simulink model "hw2_SISO_2_3_chann_final"  (R2023b)
settings: Solver=ode15s  StartTime=0.0  StopTime=4  FixedStep=0.001  RelTol=1e-3
values from neighbouring files (symbols this model uses):
  A = 1    [hw1_four_channel_bilateral_teleoperation_params.m]    (also in hw2_2_3_channel_bilateral_teleoperation_params.m; hw3_scattering_teleop_FP_params.m = 1.5; hw3_scattering_teleop_PP_params.m; hw4_tank_FP_params.m)
  Be = 100    [hw1_four_channel_bilateral_teleoperation_params.m]    (also in hw2_2_3_channel_bilateral_teleoperation_params.m; hw3_scattering_teleop_FP_params.m; hw3_scattering_teleop_PP_params.m; hw4_tank_FP_params.m)
  Bh = 1    [hw1_four_channel_bilateral_teleoperation_params.m]    (also in hw2_2_3_channel_bilateral_teleoperation_params.m; hw3_scattering_teleop_FP_params.m; hw3_scattering_teleop_PP_params.m; hw4_tank_FP_params.m)
  Bm = 20*0.8    (= 16)    [hw1_four_channel_bilateral_teleoperation_params.m]    (also in hw2_2_3_channel_bilateral_teleoperation_params.m; hw3_scattering_teleop_FP_params.m; hw3_scattering_teleop_PP_params.m; hw4_tank_FP_params.m = 32)
  Bs = 4*Bm    (= 64)    [hw1_four_channel_bilateral_teleoperation_params.m]    (also in hw2_2_3_channel_bilateral_teleoperation_params.m; hw3_scattering_teleop_FP_params.m; hw3_scattering_teleop_PP_params.m; hw4_tank_FP_params.m = 128)
  d = 0.02    [hw2_2_3_channel_bilateral_teleoperation_params.m]    (also in hw3_scattering_teleop_FP_params.m = 10; hw3_scattering_teleop_PP_params.m = 10; hw4_tank_FP_params.m = 10; hw4_tank_PP_params.m = 10)
  Dh = 20*0.8    (= 16)    [hw1_four_channel_bilateral_teleoperation_params.m]    (also in hw2_2_3_channel_bilateral_teleoperation_params.m; hw3_scattering_teleop_FP_params.m; hw3_scattering_teleop_PP_params.m; hw4_tank_FP_params.m)
  Dm = 0    [hw1_four_channel_bilateral_teleoperation_params.m]    (also in hw2_2_3_channel_bilateral_teleoperation_params.m; hw3_scattering_teleop_FP_params.m = 5; hw3_scattering_teleop_PP_params.m; hw4_tank_FP_params.m)
  Ds = 0    [hw1_four_channel_bilateral_teleoperation_params.m]    (also in hw2_2_3_channel_bilateral_teleoperation_params.m; hw3_scattering_teleop_FP_params.m; hw3_scattering_teleop_PP_params.m; hw4_tank_FP_params.m)
  Fc = 1    [hw1_four_channel_bilateral_teleoperation_params.m]    (also in hw2_2_3_channel_bilateral_teleoperation_params.m; hw3_scattering_teleop_FP_params.m; hw3_scattering_teleop_PP_params.m; hw4_tank_FP_params.m)
  Flp = 0.5    [hw1_four_channel_bilateral_teleoperation_params.m]    (also in hw2_2_3_channel_bilateral_teleoperation_params.m; hw3_scattering_teleop_FP_params.m = 0.01; hw3_scattering_teleop_PP_params.m = 0.01; hw4_tank_FP_params.m = 1)
  Jh = 1    [hw1_four_channel_bilateral_teleoperation_params.m]    (also in hw2_2_3_channel_bilateral_teleoperation_params.m; hw3_scattering_teleop_FP_params.m; hw3_scattering_teleop_PP_params.m; hw4_tank_FP_params.m)
  Ke = 200    [hw1_four_channel_bilateral_teleoperation_params.m]    (also in hw2_2_3_channel_bilateral_teleoperation_params.m; hw3_scattering_teleop_FP_params.m; hw3_scattering_teleop_PP_params.m; hw4_tank_FP_params.m)
  Km = 10*1    (= 10)    [hw1_four_channel_bilateral_teleoperation_params.m]    (also in hw2_2_3_channel_bilateral_teleoperation_params.m; hw3_scattering_teleop_FP_params.m; hw3_scattering_teleop_PP_params.m; hw4_tank_FP_params.m)
  Ks = 4*Km    (= 40)    [hw1_four_channel_bilateral_teleoperation_params.m]    (also in hw2_2_3_channel_bilateral_teleoperation_params.m; hw3_scattering_teleop_FP_params.m; hw3_scattering_teleop_PP_params.m; hw4_tank_FP_params.m)
  Mm = 0.5    [hw1_four_channel_bilateral_teleoperation_params.m]    (also in hw2_2_3_channel_bilateral_teleoperation_params.m; hw3_scattering_teleop_FP_params.m; hw3_scattering_teleop_PP_params.m; hw4_tank_FP_params.m)
  Ms = 2    [hw1_four_channel_bilateral_teleoperation_params.m]    (also in hw2_2_3_channel_bilateral_teleoperation_params.m; hw3_scattering_teleop_FP_params.m; hw3_scattering_teleop_PP_params.m; hw4_tank_FP_params.m)
  Ph = 10*1    (= 10)    [hw1_four_channel_bilateral_teleoperation_params.m]    (also in hw2_2_3_channel_bilateral_teleoperation_params.m; hw3_scattering_teleop_FP_params.m; hw3_scattering_teleop_PP_params.m; hw4_tank_FP_params.m)
  xe = 0.7    [hw1_four_channel_bilateral_teleoperation_params.m]    (also in hw2_2_3_channel_bilateral_teleoperation_params.m = 1.5; hw3_scattering_teleop_FP_params.m = 1.5; hw3_scattering_teleop_PP_params.m = 1.5; hw4_tank_FP_params.m = 1.5)
settings Model: Creator=86180  LastModifiedBy=86180

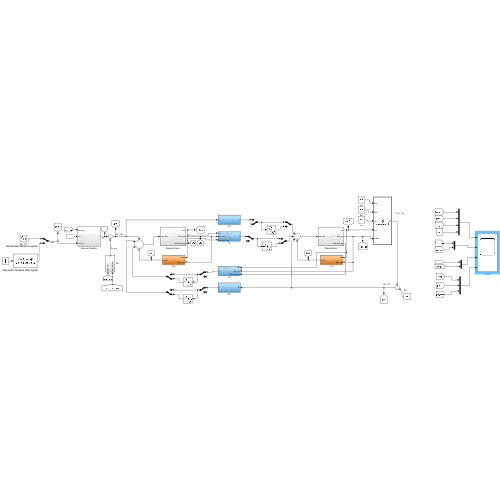
[thumbnail: Simulink's stored preview of the top-level diagram]
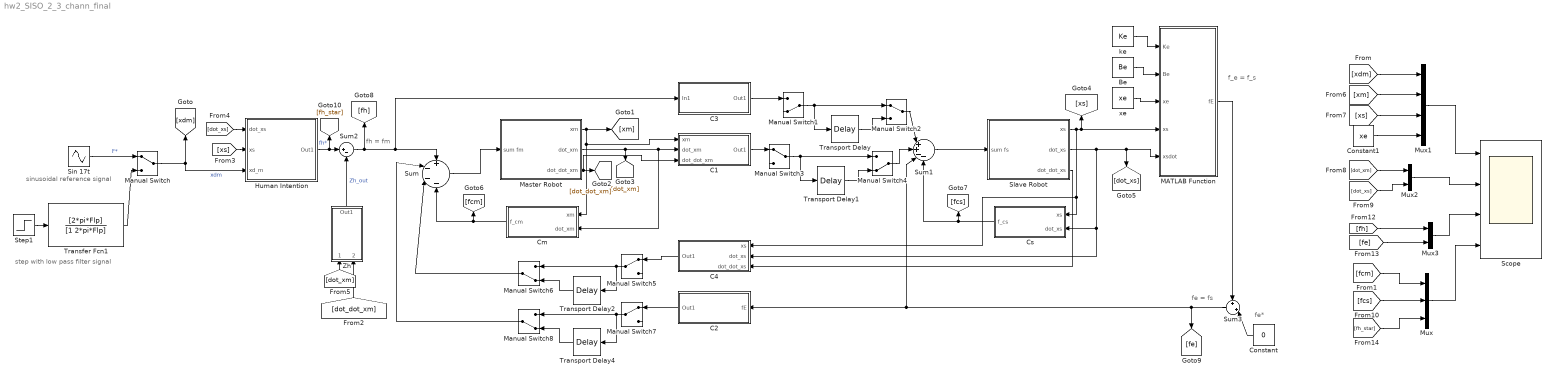
== system hw2_SISO_2_3_chann_final ==
  note: f_e = f_s
  note: fe*
  note: fe = fs
  note: fh = fm
  note: sinusoidal reference signal
  note: step with low pass filter signal
  Be : Constant  Value=Be
  C1 : Subsystem
  C2 : Subsystem
  C3 : Subsystem
  C4 : Subsystem
  Cm : Subsystem
  Constant : Constant  Value=0
  Constant1 : Constant  Value=xe
  Cs : Subsystem
  Human Intention : Subsystem
  MATLAB Function : MATLAB Function  TreatAsAtomicUnit=on
  Manual Switch{,2..3,5,7} (5 alike) : ManualSwitch
  Manual Switch{1,4,6,8} (4 alike) : ManualSwitch  CurrentSetting=0
  Master Robot : Subsystem
  Mux : Mux  Inputs=3
  Mux1 : Mux
  Mux2 : Mux  Inputs=2
  Mux3 : Mux  Inputs=2
  Scope : Scope  NumInputPorts=4
  Sin 17t : Sin  Amplitude=A  Frequency=2*pi*Fc  SampleTime=0
  Slave Robot : Subsystem
  Step1 : Step  Time=0.5  After=A  SampleTime=0
  Sum : Sum  Inputs=+---
  Sum1 : Sum  Inputs=|++--
  Sum2 : Sum  Inputs=|+-
  Sum3 : Sum  Inputs=+|+|
  Transfer Fcn1 : TransferFcn  Numerator=[2*pi*Flp]  Denominator=[1 2*pi*Flp]
  Transport Delay{,1..2,4} (4 alike) : TransportDelay  DelayTime=d
  Zh : Subsystem
  ke : Constant  Value=Ke
  xe : Constant  Value=xe
  wires:
  Manual Switch/1 -> Human Intention/3(xd_m), [xdm]  "xdm"
  Zh/1(Out1) -> Sum2/2  "Zh_out"
  Transfer Fcn1/1 -> Manual Switch/2
  Human Intention/1(Out1) -> [fh_star], Sum2/1  "fh*"
  Sin 17t/1 -> Manual Switch/1  "F*"
  Step1/1 -> Transfer Fcn1/1
  ke/1 -> MATLAB Function/1(Ke)
  xe/1 -> MATLAB Function/3(xe)
  Slave Robot/1(xs) -> Cs/1(xs), C4/1(xs), MATLAB Function/4(xs), [xs]
  MATLAB Function/1(fE) -> Sum3/1
  Be/1 -> MATLAB Function/2(Be)
  Sum2/1 -> C3/1(In1), Sum/1, [fh]
  Master Robot/2(dot_xm) -> [dot_xm], C1/2(dot_xm), Cm/2(dot_xm)
  Cm/1(f_cm) -> [fcm], Sum/4
  Slave Robot/2(dot_xs) -> Cs/2(dot_xs), C4/2(dot_xs), [dot_xs], MATLAB Function/5(xsdot)
  Cs/1(f_cs) -> [fcs], Sum1/4
  Sum3/1 -> [fe], C2/1(fE), Sum1/3
  Constant/1 -> Sum3/2
  Master Robot/1(xm) -> C1/1(xm), Cm/1(xm), [xm]
  Master Robot/3(dot_dot_xm) -> C1/3(dot_dot_xm), [dot_dot_xm]
  [dot_dot_xm] -> Zh/2(dot_dot_xm)
  [xs] -> Human Intention/2(xs)
  [dot_xs] -> Human Intention/1(dot_xs)
  Sum/1 -> Master Robot/1(sum fm)
  [dot_xm] -> Zh/1(dot_xm)
  Sum1/1 -> Slave Robot/1(sum fs)
  Slave Robot/3(dot_dot_xs) -> C4/3(dot_dot_xs)
  Mux1/1 -> Scope/1
  Constant1/1 -> Mux1/4
  [fh] -> Mux3/1
  [dot_xs] -> Mux2/2
  Mux3/1 -> Scope/3
  [fe] -> Mux3/2
  [xm] -> Mux1/2
  [fcm] -> Mux/1
  [dot_xm] -> Mux2/1
  [fcs] -> Mux/2
  [xs] -> Mux1/3
  Mux2/1 -> Scope/2
  [xdm] -> Mux1/1
  Mux/1 -> Scope/4
  [fh_star] -> Mux/3
  Transport Delay/1 -> Manual Switch2/2
  C3/1(Out1) -> Manual Switch1/1
  Manual Switch1/1 -> Transport Delay/1, Manual Switch2/1
  Manual Switch2/1 -> Sum1/1
  Manual Switch3/1 -> Transport Delay1/1, Manual Switch4/1
  C1/1(Out1) -> Manual Switch3/1
  Transport Delay1/1 -> Manual Switch4/2
  Manual Switch4/1 -> Sum1/2
  Transport Delay2/1 -> Manual Switch6/2
  Manual Switch6/1 -> Sum/3
  Manual Switch5/1 -> Transport Delay2/1, Manual Switch6/1
  C4/1(Out1) -> Manual Switch5/1
  C2/1(Out1) -> Manual Switch7/1
  Manual Switch7/1 -> Transport Delay4/1, Manual Switch8/1
  Manual Switch8/1 -> Sum/2
  Transport Delay4/1 -> Manual Switch8/2

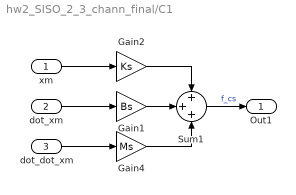
== system hw2_SISO_2_3_chann_final/C1 ==
  xm : Inport
  dot_xm : Inport  Port=2
  dot_dot_xm : Inport  Port=3
  Gain1 : Gain  Gain=Bs
  Gain2 : Gain  Gain=Ks
  Gain4 : Gain  Gain=Ms
  Sum1 : Sum  Inputs=+++
  Out1 : Outport
  wires:
  dot_xm/1 -> Gain1/1
  Gain1/1 -> Sum1/2
  dot_dot_xm/1 -> Gain4/1
  xm/1 -> Gain2/1
  Sum1/1 -> Out1/1  "f_cs"
  Gain2/1 -> Sum1/1
  Gain4/1 -> Sum1/3

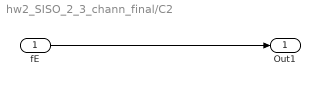
== system hw2_SISO_2_3_chann_final/C2 ==
  fE : Inport
  Out1 : Outport
  wires:
  fE/1 -> Out1/1

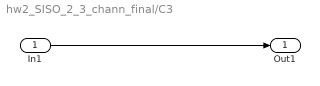
== system hw2_SISO_2_3_chann_final/C3 ==
  In1 : Inport
  Out1 : Outport
  wires:
  In1/1 -> Out1/1

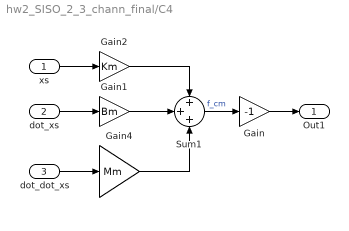
== system hw2_SISO_2_3_chann_final/C4 ==
  xs : Inport
  dot_xs : Inport  Port=2
  dot_dot_xs : Inport  Port=3
  Gain : Gain  Gain=-1
  Gain1 : Gain  Gain=Bm
  Gain2 : Gain  Gain=Km
  Gain4 : Gain  Gain=Mm
  Sum1 : Sum  Inputs=+++
  Out1 : Outport
  wires:
  Sum1/1 -> Gain/1  "f_cm"
  xs/1 -> Gain2/1
  dot_dot_xs/1 -> Gain4/1
  Gain1/1 -> Sum1/2
  Gain2/1 -> Sum1/1
  dot_xs/1 -> Gain1/1
  Gain4/1 -> Sum1/3
  Gain/1 -> Out1/1

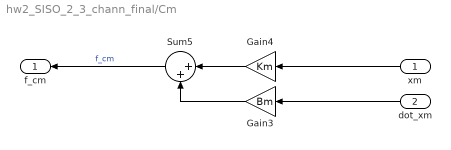
== system hw2_SISO_2_3_chann_final/Cm ==
  xm : Inport
  dot_xm : Inport  Port=2
  Gain3 : Gain  Gain=Bm
  Gain4 : Gain  Gain=Km
  Sum5 : Sum  Inputs=|++
  f_cm : Outport
  wires:
  Sum5/1 -> f_cm/1  "f_cm"
  Gain4/1 -> Sum5/1
  dot_xm/1 -> Gain3/1
  Gain3/1 -> Sum5/2
  xm/1 -> Gain4/1

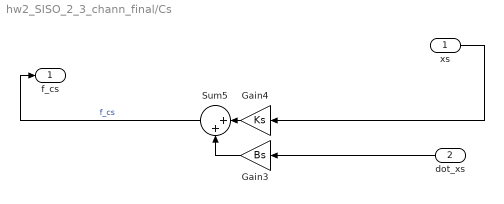
== system hw2_SISO_2_3_chann_final/Cs ==
  xs : Inport
  dot_xs : Inport  Port=2
  Gain3 : Gain  Gain=Bs
  Gain4 : Gain  Gain=Ks
  Sum5 : Sum  Inputs=|++
  f_cs : Outport
  wires:
  dot_xs/1 -> Gain3/1
  Sum5/1 -> f_cs/1  "f_cs"
  xs/1 -> Gain4/1
  Gain3/1 -> Sum5/2
  Gain4/1 -> Sum5/1

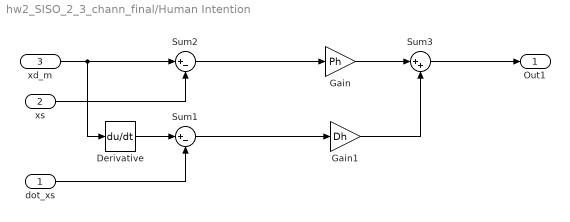
== system hw2_SISO_2_3_chann_final/Human Intention ==
  dot_xs : Inport
  xs : Inport  Port=2
  xd_m : Inport  Port=3
  Derivative : Derivative
  Gain : Gain  Gain=Ph
  Gain1 : Gain  Gain=Dh
  Sum1 : Sum  Inputs=|+-
  Sum2 : Sum  Inputs=|+-
  Sum3 : Sum  Inputs=|++
  Out1 : Outport
  wires:
  xs/1 -> Sum2/2
  dot_xs/1 -> Sum1/2
  Sum2/1 -> Gain/1
  Sum1/1 -> Gain1/1
  Gain1/1 -> Sum3/2
  Gain/1 -> Sum3/1
  Sum3/1 -> Out1/1
  xd_m/1 -> Derivative/1, Sum2/1
  Derivative/1 -> Sum1/1

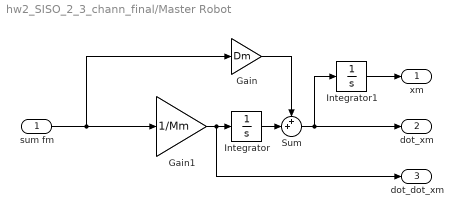
== system hw2_SISO_2_3_chann_final/Master Robot ==
  sum fm : Inport
  Gain : Gain  Gain=Dm
  Gain1 : Gain  Gain=1/Mm
  Integrator : Integrator
  Integrator1 : Integrator
  Sum : Sum  Inputs=++|
  xm : Outport
  dot_xm : Outport  Port=2
  dot_dot_xm : Outport  Port=3
  wires:
  Gain/1 -> Sum/1
  Integrator1/1 -> xm/1
  Integrator/1 -> Sum/2
  sum fm/1 -> Gain/1, Gain1/1
  Gain1/1 -> dot_dot_xm/1, Integrator/1
  Sum/1 -> dot_xm/1, Integrator1/1

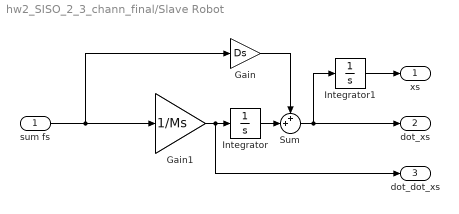
== system hw2_SISO_2_3_chann_final/Slave Robot ==
  sum fs : Inport
  Gain : Gain  Gain=Ds
  Gain1 : Gain  Gain=1/Ms
  Integrator : Integrator
  Integrator1 : Integrator
  Sum : Sum  Inputs=++|
  xs : Outport
  dot_xs : Outport  Port=2
  dot_dot_xs : Outport  Port=3
  wires:
  Integrator1/1 -> xs/1
  Gain1/1 -> dot_dot_xs/1, Integrator/1
  Gain/1 -> Sum/1
  sum fs/1 -> Gain/1, Gain1/1
  Integrator/1 -> Sum/2
  Sum/1 -> Integrator1/1, dot_xs/1

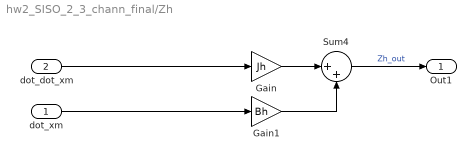
== system hw2_SISO_2_3_chann_final/Zh ==
  dot_xm : Inport
  dot_dot_xm : Inport  Port=2
  Gain : Gain  Gain=Jh
  Gain1 : Gain  Gain=Bh
  Sum4 : Sum  Inputs=|++
  Out1 : Outport
  wires:
  dot_dot_xm/1 -> Gain/1
  Gain1/1 -> Sum4/2
  Gain/1 -> Sum4/1
  Sum4/1 -> Out1/1  "Zh_out"
  dot_xm/1 -> Gain1/1

== matlab function hw2_SISO_2_3_chann_final/MATLAB Function ==
  data: Ke input; fE output; Be input; xe input; xs input; xsdot input
function fE = environment(Ke, Be, xe, xs, xsdot)
    if xs > xe
        fE = Ke * (xs - xe) + Be * xsdot; % Plot both contributions Ke and Be
    else
        fE = 0;
    end
end
